simulink model "ORC_physical_modified"  (R2017a)
settings: Solver=VariableStepAuto  StartTime=0.0  StopTime=10.0  RelTol=1e-3
undefined symbols (not defined in the file): L_init, pipe_area, Throttle_param
libraries: fl_lib x16, nesl_utility x5, RankineCycle_lib x3
(part 3 of 5)

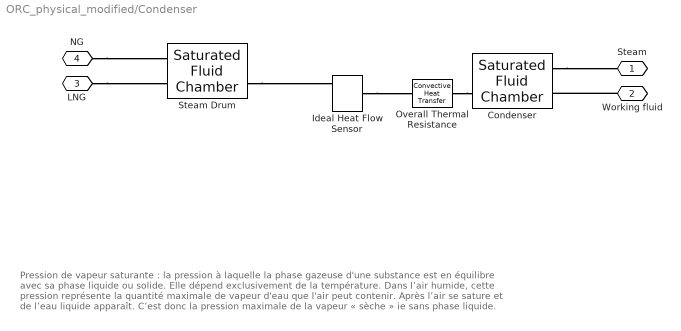
== system ORC_physical_modified/Condenser ==
  note: Pression de vapeur saturante : la pression à laquelle la phase gazeuse d'une substance est en équilibre avec sa phase liquide ou solide. Elle dépend exclusivement de la température. Dans l’air humide,
      | cette pression représente la quantité maximale de vapeur d'eau que l'air peut contenir. Après l’air se sature et de l’eau liquide apparaît. C’est donc la pression maximale de la vapeur « sèche » ie sans phase liquide.
  Condenser : RankineCycle_lib/Saturated Fluid Chamber  volume=0.5 m^3  area_A=0.01 m^2  area_B=0.01 m^2  L_min=0.01  L_max=0.99  p_I_specify=on  p_I_priority=High  p_I=p_init MPa  p_I_nominal_specify=off  p_I_nominal_unit=MPa  p_I_nominal_value=1  L_specify=on  L_priority=High  L=L_init  L_nominal_specify=off  L_nominal_unit=1  L_nominal_value=1
  Ideal Heat Flow Sensor : fl_lib/Thermal/Thermal Sensors/Ideal Heat Flow Sensor
      settings: SourceProductName=Foundation Library
  Overall Thermal Resistance : fl_lib/Thermal/Thermal Elements/Convective Heat Transfer  area=condenser_area m^2  heat_tr_coeff=condenser_heat_coeff W/(m^2 * K)  Q_specify=off  Q_priority=None  Q=0 J/s  Q_nominal_specify=off  Q_nominal_unit=J/s  Q_nominal_value=1  T_specify=off  T_priority=None  T=0 K  T_nominal_specify=off  T_nominal_unit=K  T_nominal_value=1
      settings: SourceProductName=Foundation Library
  Steam Drum : RankineCycle_lib/Saturated Fluid Chamber  volume=0.5 m^3  area_A=0.01 m^2  area_B=0.01 m^2  L_min=0.01  L_max=0.99  p_I_specify=on  p_I_priority=High  p_I=p_init MPa  p_I_nominal_specify=off  p_I_nominal_unit=MPa  p_I_nominal_value=1  L_specify=on  L_priority=High  L=1  L_nominal_specify=off  L_nominal_unit=1  L_nominal_value=1
  Steam : PMIOPort  Port=1  Side=Right
  Working fluid : PMIOPort  Port=2  Side=Left
  LNG : PMIOPort  Port=3  Side=Left
  NG : PMIOPort  Port=4  Side=Right
  connections:
  Steam Drum/RConn2 -- Ideal Heat Flow Sensor/RConn2
  Ideal Heat Flow Sensor/LConn1 -- Overall Thermal Resistance/LConn1
  Condenser/LConn1 -- Steam/RConn1
  Working fluid/RConn1 -- Condenser/LConn2
  Overall Thermal Resistance/RConn1 -- Condenser/RConn2
  LNG/RConn1 -- Steam Drum/LConn2
  NG/RConn1 -- Steam Drum/LConn1

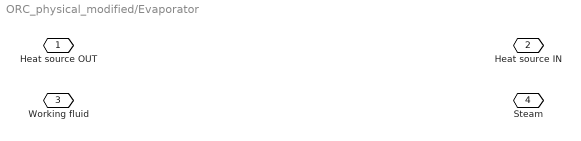
== system ORC_physical_modified/Evaporator ==
  Heat source OUT : PMIOPort  Port=1  Side=Left
  Heat source IN : PMIOPort  Port=2  Side=Right
  Working fluid : PMIOPort  Port=3  Side=Left
  Steam : PMIOPort  Port=4  Side=Right

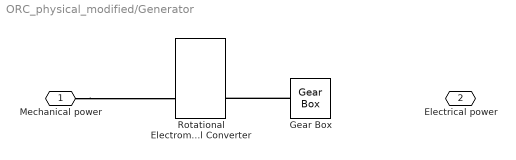
== system ORC_physical_modified/Generator ==
  Gear Box : fl_lib/Mechanical/Mechanisms/Gear Box  ratio=5  t_in_specify=off  t_in_priority=None  t_in=0 N*m  t_in_nominal_specify=off  t_in_nominal_unit=N*m  t_in_nominal_value=1  t_out_specify=off  t_out_priority=None  t_out=0 N*m  t_out_nominal_specify=off  t_out_nominal_unit=N*m  t_out_nominal_value=1
  Rotational Electromechanical Converter : fl_lib/Electrical/Electrical Elements/Rotational Electromechanical Converter  K=0.1 V/(rad/s)  i_specify=off  i_priority=None  i=0 A  i_nominal_specify=off  i_nominal_unit=A  i_nominal_value=1  v_specify=off  v_priority=None  v=0 V  v_nominal_specify=off  v_nominal_unit=V  v_nominal_value=1  t_specify=off  t_priority=None  t=0 N*m  t_nominal_specify=off  t_nominal_unit=N*m  t_nominal_value=1  w_specify=off  w_priority=None  w=0 rad/s  w_nominal_specify=off  w_nominal_unit=rad/s  w_nominal_value=1
      settings: SourceProductName=Simscape
  Mechanical power : PMIOPort  Port=1  Side=Left
  Electrical power : PMIOPort  Port=2  Side=Right
  connections:
  Mechanical power/RConn1 -- Rotational Electromechanical Converter/RConn2
  Gear Box/LConn1 -- Rotational Electromechanical Converter/LConn2
